simulink subsystem "Day1_Scenario_2"  (R2024a)
settings: Solver=VariableStepAuto  StartTime=0.0  StopTime=10.0  RelTol=1e-3
libraries: CarMaker4SL x2
settings Model: Creator=junhyung.cha  LastModifiedBy=User

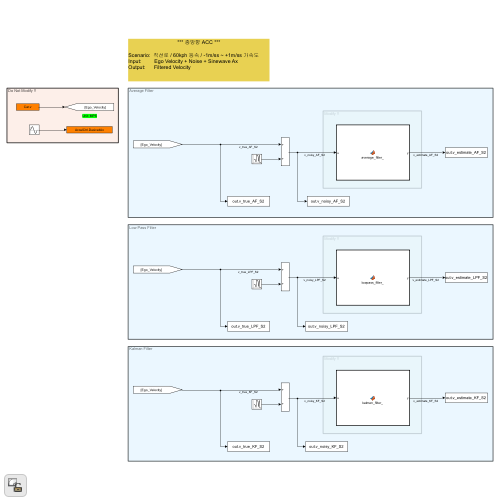
[thumbnail: Simulink's stored preview of the top-level diagram]
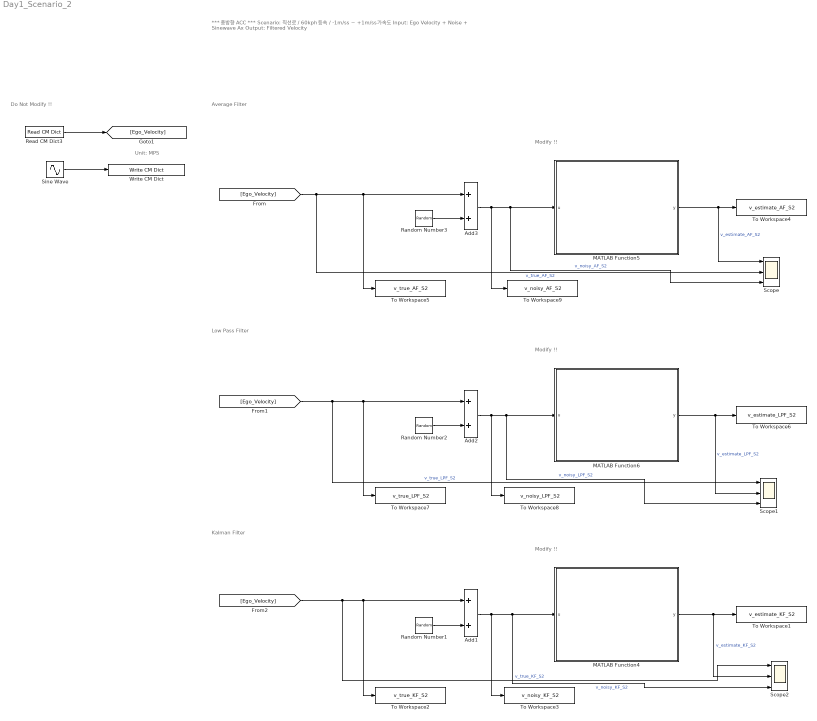
== system Day1_Scenario_2 ==
  note: Do Not Modify !!
  note: Low Pass Filter
  note: Average Filter
  note: Modify !!
  note: Modify !!
  note: Kalman Filter
  note: Modify !!
  note: *** 종방향 ACC ***
      |
      | Scenario: 직선로 / 60kph 등속 / -1m/ss ~ +1m/ss 가속도
      | Input: Ego Velocity + Noise + Sinewave Ax
      | Output: Filtered Velocity
  note: Unit: MPS
  Add1 : Sum
  Add2 : Sum
  Add3 : Sum
  MATLAB Function4 : MATLAB Function  TreatAsAtomicUnit=on
  MATLAB Function5 : MATLAB Function  TreatAsAtomicUnit=on
  MATLAB Function6 : MATLAB Function  TreatAsAtomicUnit=on
  Random Number1 : RandomNumber
  Random Number2 : RandomNumber
  Random Number3 : RandomNumber
  Read CM Dict3 : CarMaker4SL/Read CM Dict  xname=Car.v  xsync=off  xstime=Inherited
  Scope : Scope  NumInputPorts=3
  Scope1 : Scope  NumInputPorts=3
  Scope2 : Scope  NumInputPorts=3
  Sine Wave : Sin
  To Workspace1 : ToWorkspace  VariableName=v_estimate_KF_S2  SaveFormat=Timeseries  SampleTime=-1
  To Workspace2 : ToWorkspace  VariableName=v_true_KF_S2  SaveFormat=Timeseries  SampleTime=-1
  To Workspace3 : ToWorkspace  VariableName=v_noisy_KF_S2  SaveFormat=Timeseries  SampleTime=-1
  To Workspace4 : ToWorkspace  VariableName=v_estimate_AF_S2  SaveFormat=Timeseries  SampleTime=-1
  To Workspace5 : ToWorkspace  VariableName=v_true_AF_S2  SaveFormat=Timeseries  SampleTime=-1
  To Workspace6 : ToWorkspace  VariableName=v_estimate_LPF_S2  SaveFormat=Timeseries  SampleTime=-1
  To Workspace7 : ToWorkspace  VariableName=v_true_LPF_S2  SaveFormat=Timeseries  SampleTime=-1
  To Workspace8 : ToWorkspace  VariableName=v_noisy_LPF_S2  SaveFormat=Timeseries  SampleTime=-1
  To Workspace9 : ToWorkspace  VariableName=v_noisy_AF_S2  SaveFormat=Timeseries  SampleTime=-1
  Write CM Dict : CarMaker4SL/Write CM Dict  xname=AccelCtrl.DesiredAx  xsync=off
  wires:
  Sine Wave/1 -> Write CM Dict/1
  Random Number3/1 -> Add3/2
  Add3/1 -> To Workspace9/1, MATLAB Function5/1(u), Scope/3  "v_noisy_AF_S2"
  Add2/1 -> To Workspace8/1, MATLAB Function6/1(u), Scope1/3  "v_noisy_LPF_S2"
  [Ego_Velocity] -> Add2/1, To Workspace7/1, Scope1/1  "v_true_LPF_S2"
  MATLAB Function6/1(y) -> To Workspace6/1, Scope1/2  "v_estimate_LPF_S2"
  Random Number2/1 -> Add2/2
  MATLAB Function5/1(y) -> To Workspace4/1, Scope/1  "v_estimate_AF_S2"
  Add1/1 -> To Workspace3/1, MATLAB Function4/1(u), Scope2/3  "v_noisy_KF_S2"
  [Ego_Velocity] -> Add1/1, To Workspace2/1, Scope2/1  "v_true_KF_S2"
  MATLAB Function4/1(y) -> To Workspace1/1, Scope2/2  "v_estimate_KF_S2"
  [Ego_Velocity] -> Add3/1, To Workspace5/1, Scope/2  "v_true_AF_S2"
  Random Number1/1 -> Add1/2
  Read CM Dict3/1 -> [Ego_Velocity]

== matlab function Day1_Scenario_2/MATLAB Function5 ==
  settings: updateMethod=DISCRETE  sampleTime=0.05
  data: u input; y output
function y = average_filter_(u)
    y = 0;
    %#codegen
    % 누적 합(sum)과 카운트(count)를 persistent로 유지
    
    persistent sum count
    if isempty(sum)
      sum   = 0;
      count = 0;
    end
    
    % 업데이트
    sum   = sum + u;
    count = count + 1;
    
    % 출력: 누적 평균
    y = sum / count;
end

== matlab function Day1_Scenario_2/MATLAB Function6 ==
  settings: updateMethod=DISCRETE  sampleTime=0.05
  data: u input; y output
function y = lowpass_filter_(u)
    y = 0;
    %#codegen
    % y[n] = alpha*u[n] + (1-alpha)*y[n-1]
    
    persistent alpha y_prev
    if isempty(alpha)
      alpha  = 0.2;    % Python 예제의 alpha
      y_prev = u;      % 초기 출력
    end
    
    % 지수 이동 평균
    y      = alpha*u + (1-alpha)*y_prev;
    y_prev = y;       % 상태 갱신
end

== matlab function Day1_Scenario_2/MATLAB Function4 ==
  settings: updateMethod=DISCRETE  sampleTime=0.05
  data: u input; y output
function y = kalman_filter_(u)
    y = 0;
%#codegen
% u : [측정값; 제어입력] 또는 스칼라(측정값만)
% y : 칼만 필터가 추정한 속도

  persistent A B C Q R P x_prev dt
  if isempty(A)
    % 1) Python 코드와 같은 파라미터로 초기화
    dt      = 0.1;    % step_time
    A       = 1.0;    % 상태 전이
    B       = dt;     % Python에서 B=step_time
    C       = 1.0;    % 관측 계수
    Q       = 0.01;   % 프로세스 잡음 분산
    R       = 1.0;    % 측정 잡음 분산
    P       = 10.0;   % 초기 오차 공분산
    x_prev  = u(1);   % 초기 상태 추정치: 첫 측정값
  end
  

  % 2) 입력 분리
  if numel(u) >= 2
    z       = u(1);  % 측정값
    input_u = u(2);  % 제어입력(가속도)
  else
    z       = u;     % 스칼라만 들어온 경우
    input_u = 0;     % 제어입력이 없으면 0
  end



  % — Prediction 단계 —
  x_pred = A * x_prev + B * input_u;
  P_pred = A * P * A + Q;

  % — Update 단계 —
  K      = P_pred * C / (C * P_pred * C + R);
  x_est  = x_pred + K * (z - C * x_pred);
  P      = (1 - K * C) * P_pred;

  % — 출력 및 내부 상태 저장 —
  y      = x_est;   % 블록 출력
  x_prev = x_est;   % 다음 스텝 예측을 위한 저장
end
